simulink library "tramontina_database_curtislib"  (R2023a)
settings: Solver=VariableStepAuto  StartTime=0.0  StopTime=10.0  RelTol=1e-3
libraries: canmsglib x22, simulink x1
settings Model: Creator=matlab.cut  LastModifiedBy=matlab.cut

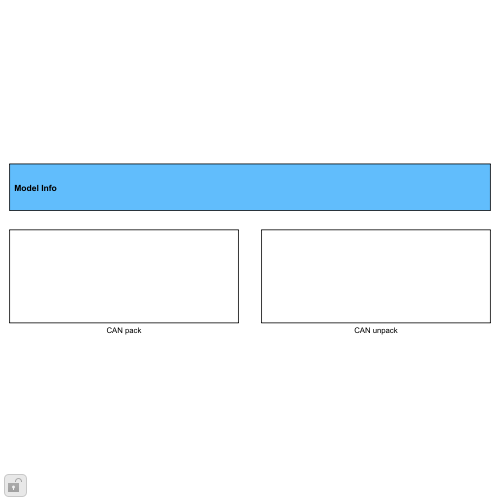
[thumbnail: Simulink's stored preview of the top-level diagram]
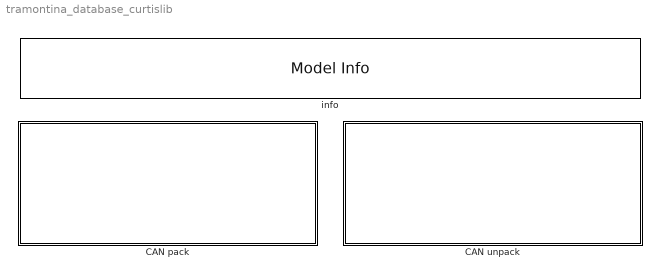
== system tramontina_database_curtislib ==
  CAN pack : Subsystem
  CAN unpack : Subsystem
  info : simulink/Model-Wide Utilities/Model Info  Frame=on  DisplayStringWithTags=SPEEDGOAT CAN Database Library for: tramontina_database_curtis  HorizontalTextAlignment=Left  LeftAlignmentValue=0.01

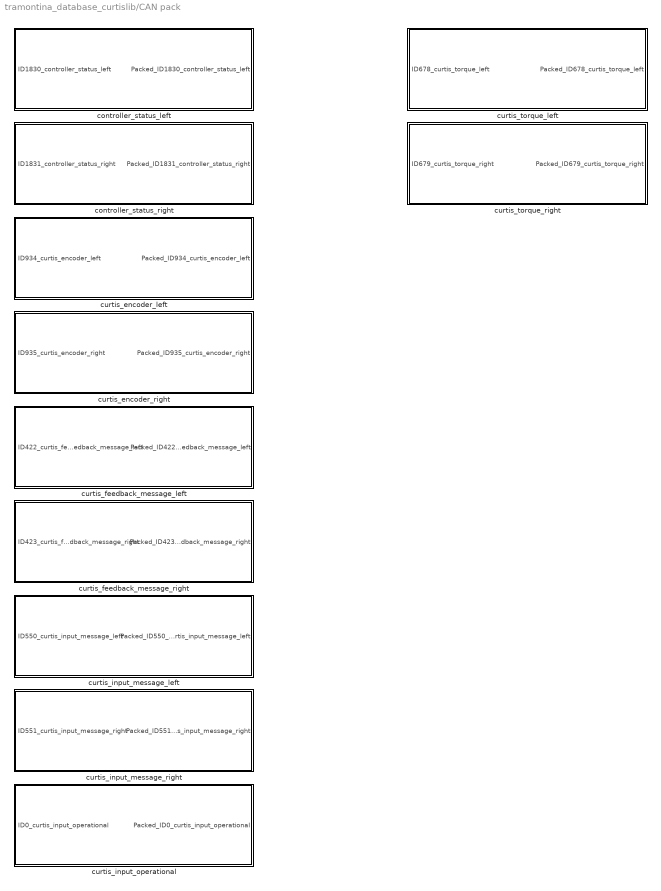
== system tramontina_database_curtislib/CAN pack ==
  controller_status_left : Subsystem
  controller_status_right : Subsystem
  curtis_encoder_left : Subsystem
  curtis_encoder_right : Subsystem
  curtis_feedback_message_left : Subsystem
  curtis_feedback_message_right : Subsystem
  curtis_input_message_left : Subsystem
  curtis_input_message_right : Subsystem
  curtis_input_operational : Subsystem
  curtis_torque_left : Subsystem
  curtis_torque_right : Subsystem

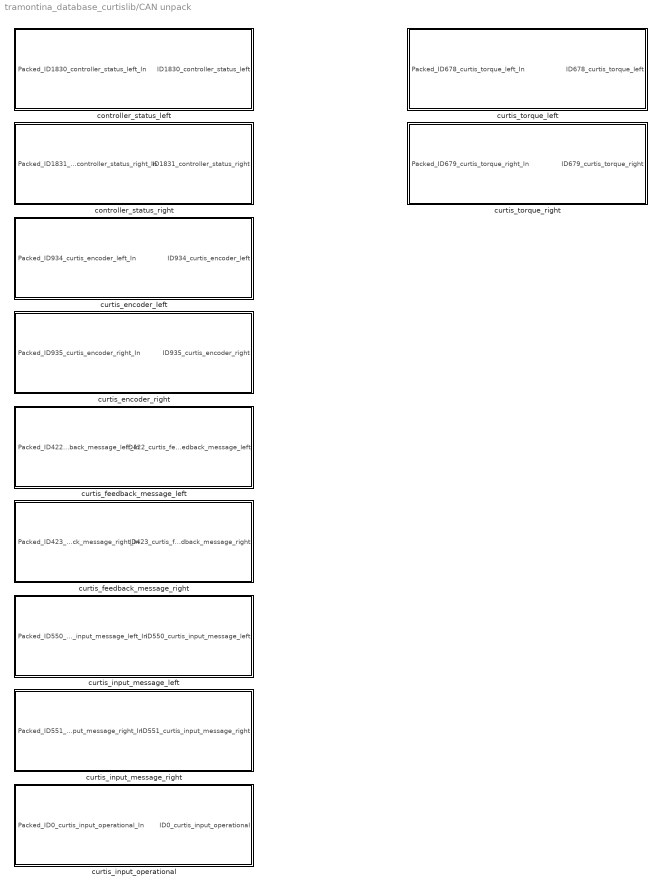
== system tramontina_database_curtislib/CAN unpack ==
  controller_status_left : Subsystem
  controller_status_right : Subsystem
  curtis_encoder_left : Subsystem
  curtis_encoder_right : Subsystem
  curtis_feedback_message_left : Subsystem
  curtis_feedback_message_right : Subsystem
  curtis_input_message_left : Subsystem
  curtis_input_message_right : Subsystem
  curtis_input_operational : Subsystem
  curtis_torque_left : Subsystem
  curtis_torque_right : Subsystem

== system tramontina_database_curtislib/CAN pack/controller_status_left ==
  In Bus Element : Inport  PortName=ID1830_controller_status_left  Element=controller_mode_left
  controller_status_left : canmsglib/CAN Pack  CANdbFile=C:\Users\matlab.cut\Desktop\matlab\dev_interno_tramontina-main\AGV-Dev-Simulink\Docs\tramontina_database_curtis.dbc  MsgList=controller_status_left  MsgName=controller_status_left  MsgIDType=Standard (11-bit identifier)  MsgIdentifier=1830  MsgLength=1  Remote=off  ApplyMinMax=off  BusOutput=on  SignalInfo={'controller_mode_left','0','8','LE','unsigned','Standard','0','1','0','0','255'}
      settings: DataFormat=manually specified signals
  Packed_ID1830_controller_status_left : Outport
  wires:
  controller_status_left/1 -> Packed_ID1830_controller_status_left/1
  In Bus Element/1 -> controller_status_left/1

== system tramontina_database_curtislib/CAN pack/controller_status_right ==
  In Bus Element : Inport  PortName=ID1831_controller_status_right  Element=controller_mode_right
  controller_status_right : canmsglib/CAN Pack  CANdbFile=C:\Users\matlab.cut\Desktop\matlab\dev_interno_tramontina-main\AGV-Dev-Simulink\Docs\tramontina_database_curtis.dbc  MsgList=controller_status_right  MsgName=controller_status_right  MsgIDType=Standard (11-bit identifier)  MsgIdentifier=1831  MsgLength=1  Remote=off  ApplyMinMax=off  BusOutput=on  SignalInfo={'controller_mode_right','0','8','LE','unsigned','Standard','0','1','0','0','255'}
      settings: DataFormat=manually specified signals
  Packed_ID1831_controller_status_right : Outport
  wires:
  controller_status_right/1 -> Packed_ID1831_controller_status_right/1
  In Bus Element/1 -> controller_status_right/1

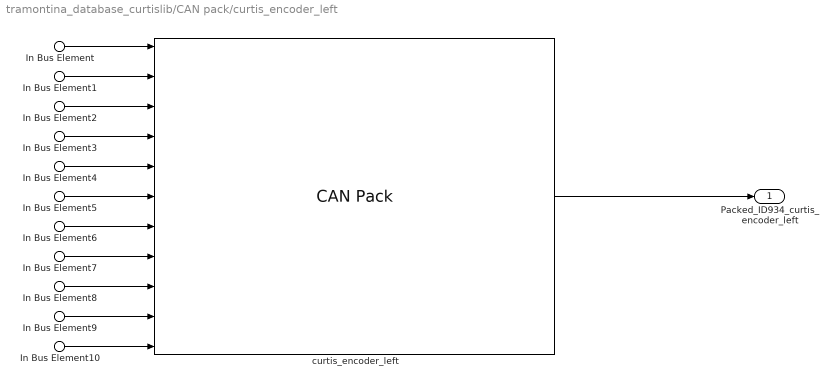
== system tramontina_database_curtislib/CAN pack/curtis_encoder_left ==
  In Bus Element : Inport  PortName=ID934_curtis_encoder_left  Element=rotor_position_left
  In Bus Element1 : Inport  PortName=ID934_curtis_encoder_left  Element=switch1
  In Bus Element2 : Inport  PortName=ID934_curtis_encoder_left  Element=switch10
  In Bus Element3 : Inport  PortName=ID934_curtis_encoder_left  Element=switch12
  In Bus Element4 : Inport  PortName=ID934_curtis_encoder_left  Element=switch13
  In Bus Element5 : Inport  PortName=ID934_curtis_encoder_left  Element=switch15
  In Bus Element6 : Inport  PortName=ID934_curtis_encoder_left  Element=switch18
  In Bus Element7 : Inport  PortName=ID934_curtis_encoder_left  Element=switch6
  In Bus Element8 : Inport  PortName=ID934_curtis_encoder_left  Element=switch7
  In Bus Element9 : Inport  PortName=ID934_curtis_encoder_left  Element=switch8
  In Bus Element10 : Inport  PortName=ID934_curtis_encoder_left  Element=switch9
  curtis_encoder_left : canmsglib/CAN Pack  CANdbFile=C:\Users\matlab.cut\Desktop\matlab\dev_interno_tramontina-main\AGV-Dev-Simulink\Docs\tramontina_database_curtis.dbc  MsgList=curtis_encoder_left  MsgName=curtis_encoder_left  MsgIDType=Standard (11-bit identifier)  MsgIdentifier=934  MsgLength=8  Remote=off  ApplyMinMax=off  BusOutput=on  SignalInfo={'rotor_position_left','0','32','LE','signed','Standard','0','0.00024414','0','-524288','524287';'switch1','32','1','LE','unsigned','Standard','0','1','0','0','1';'switch10','41','1','LE','unsigned','Standard','0','1','0','0','1';'switch12','43','1','LE','unsigned','Standard','0','1','0','0','1';'switch13','44','1','LE','unsigned','Standard','0','1','0','0','1';'switch15','46','1','LE','unsigned','Standard','0','1','0','0','1';'switch18','49','1','LE','unsigned','Standard','0','1','0','0','1';'switch6','37','1','LE','unsigned','Standard','0','1','0','0','1';'switch7','38','1','LE','unsigned','Standard','0','1','0','0','1';'switch8','39','1','LE','unsigned','Standard','0','1','0','0','1';'switch9','40','1','LE','unsigned','Standard','0','1','0','0','1'}
      settings: DataFormat=manually specified signals
  Packed_ID934_curtis_encoder_left : Outport
  wires:
  curtis_encoder_left/1 -> Packed_ID934_curtis_encoder_left/1
  In Bus Element/1 -> curtis_encoder_left/1
  In Bus Element1/1 -> curtis_encoder_left/2
  In Bus Element2/1 -> curtis_encoder_left/3
  In Bus Element3/1 -> curtis_encoder_left/4
  In Bus Element4/1 -> curtis_encoder_left/5
  In Bus Element5/1 -> curtis_encoder_left/6
  In Bus Element6/1 -> curtis_encoder_left/7
  In Bus Element7/1 -> curtis_encoder_left/8
  In Bus Element8/1 -> curtis_encoder_left/9
  In Bus Element9/1 -> curtis_encoder_left/10
  In Bus Element10/1 -> curtis_encoder_left/11

== system tramontina_database_curtislib/CAN pack/curtis_encoder_right ==
  In Bus Element : Inport  PortName=ID935_curtis_encoder_right  Element=rotor_position_rigth
  curtis_encoder_right : canmsglib/CAN Pack  CANdbFile=C:\Users\matlab.cut\Desktop\matlab\dev_interno_tramontina-main\AGV-Dev-Simulink\Docs\tramontina_database_curtis.dbc  MsgList=curtis_encoder_right  MsgName=curtis_encoder_right  MsgIDType=Standard (11-bit identifier)  MsgIdentifier=935  MsgLength=4  Remote=off  ApplyMinMax=off  BusOutput=on  SignalInfo={'rotor_position_rigth','0','32','LE','signed','Standard','0','0.00024414','0','-524288','524287'}
      settings: DataFormat=manually specified signals
  Packed_ID935_curtis_encoder_right : Outport
  wires:
  curtis_encoder_right/1 -> Packed_ID935_curtis_encoder_right/1
  In Bus Element/1 -> curtis_encoder_right/1

== system tramontina_database_curtislib/CAN pack/curtis_feedback_message_left ==
  In Bus Element : Inport  PortName=ID422_curtis_feedback_message_left  Element=motor_current_left
  In Bus Element1 : Inport  PortName=ID422_curtis_feedback_message_left  Element=motor_rpm_left
  In Bus Element2 : Inport  PortName=ID422_curtis_feedback_message_left  Element=motor_temperature_left
  curtis_feedback_message_left : canmsglib/CAN Pack  CANdbFile=C:\Users\matlab.cut\Desktop\matlab\dev_interno_tramontina-main\AGV-Dev-Simulink\Docs\tramontina_database_curtis.dbc  MsgList=curtis_feedback_message_left  MsgName=curtis_feedback_message_left  MsgIDType=Standard (11-bit identifier)  MsgIdentifier=422  MsgLength=6  Remote=off  ApplyMinMax=off  BusOutput=on  SignalInfo={'motor_current_left','0','16','LE','unsigned','Standard','0','0.1','0','0','1000';'motor_rpm_left','16','16','LE','signed','Standard','0','1','0','-32768','32767';'motor_temperature_left','32','16','LE','signed','Standard','0','0.1','0','-100','300'}
      settings: DataFormat=manually specified signals
  Packed_ID422_curtis_feedback_message_left : Outport
  wires:
  curtis_feedback_message_left/1 -> Packed_ID422_curtis_feedback_message_left/1
  In Bus Element/1 -> curtis_feedback_message_left/1
  In Bus Element1/1 -> curtis_feedback_message_left/2
  In Bus Element2/1 -> curtis_feedback_message_left/3

== system tramontina_database_curtislib/CAN pack/curtis_feedback_message_right ==
  In Bus Element : Inport  PortName=ID423_curtis_feedback_message_right  Element=motor_current_right
  In Bus Element1 : Inport  PortName=ID423_curtis_feedback_message_right  Element=motor_rpm_right
  In Bus Element2 : Inport  PortName=ID423_curtis_feedback_message_right  Element=motor_temperature_right
  curtis_feedback_message_right : canmsglib/CAN Pack  CANdbFile=C:\Users\matlab.cut\Desktop\matlab\dev_interno_tramontina-main\AGV-Dev-Simulink\Docs\tramontina_database_curtis.dbc  MsgList=curtis_feedback_message_right  MsgName=curtis_feedback_message_right  MsgIDType=Standard (11-bit identifier)  MsgIdentifier=423  MsgLength=6  Remote=off  ApplyMinMax=off  BusOutput=on  SignalInfo={'motor_current_right','0','16','LE','unsigned','Standard','0','0.1','0','0','1000';'motor_rpm_right','16','16','LE','signed','Standard','0','1','0','-32768','32767';'motor_temperature_right','32','16','LE','signed','Standard','0','0.1','0','-100','300'}
      settings: DataFormat=manually specified signals
  Packed_ID423_curtis_feedback_message_right : Outport
  wires:
  curtis_feedback_message_right/1 -> Packed_ID423_curtis_feedback_message_right/1
  In Bus Element/1 -> curtis_feedback_message_right/1
  In Bus Element1/1 -> curtis_feedback_message_right/2
  In Bus Element2/1 -> curtis_feedback_message_right/3

== system tramontina_database_curtislib/CAN pack/curtis_input_message_left ==
  In Bus Element : Inport  PortName=ID550_curtis_input_message_left  Element=rpm_set_left
  curtis_input_message_left : canmsglib/CAN Pack  CANdbFile=C:\Users\matlab.cut\Desktop\matlab\dev_interno_tramontina-main\AGV-Dev-Simulink\Docs\tramontina_database_curtis.dbc  MsgList=curtis_input_message_left  MsgName=curtis_input_message_left  MsgIDType=Standard (11-bit identifier)  MsgIdentifier=550  MsgLength=8  Remote=off  ApplyMinMax=off  BusOutput=on  SignalInfo={'rpm_set_left','0','16','LE','signed','Standard','0','0.091553','0','-3000','3000'}
      settings: DataFormat=manually specified signals
  Packed_ID550_curtis_input_message_left : Outport
  wires:
  curtis_input_message_left/1 -> Packed_ID550_curtis_input_message_left/1
  In Bus Element/1 -> curtis_input_message_left/1

== system tramontina_database_curtislib/CAN pack/curtis_input_message_right ==
  In Bus Element : Inport  PortName=ID551_curtis_input_message_right  Element=rpm_set_right
  curtis_input_message_right : canmsglib/CAN Pack  CANdbFile=C:\Users\matlab.cut\Desktop\matlab\dev_interno_tramontina-main\AGV-Dev-Simulink\Docs\tramontina_database_curtis.dbc  MsgList=curtis_input_message_right  MsgName=curtis_input_message_right  MsgIDType=Standard (11-bit identifier)  MsgIdentifier=551  MsgLength=8  Remote=off  ApplyMinMax=off  BusOutput=on  SignalInfo={'rpm_set_right','0','16','LE','signed','Standard','0','0.091553','0','-3000','3000'}
      settings: DataFormat=manually specified signals
  Packed_ID551_curtis_input_message_right : Outport
  wires:
  curtis_input_message_right/1 -> Packed_ID551_curtis_input_message_right/1
  In Bus Element/1 -> curtis_input_message_right/1

== system tramontina_database_curtislib/CAN pack/curtis_input_operational ==
  In Bus Element : Inport  PortName=ID0_curtis_input_operational  Element=pre_operational
  curtis_input_operational : canmsglib/CAN Pack  CANdbFile=C:\Users\matlab.cut\Desktop\matlab\dev_interno_tramontina-main\AGV-Dev-Simulink\Docs\tramontina_database_curtis.dbc  MsgList=curtis_input_operational  MsgName=curtis_input_operational  MsgIDType=Standard (11-bit identifier)  MsgIdentifier=0  MsgLength=8  Remote=off  ApplyMinMax=off  BusOutput=on  SignalInfo={'pre_operational','0','8','LE','unsigned','Standard','0','1','0','-Inf','Inf'}
      settings: DataFormat=manually specified signals
  Packed_ID0_curtis_input_operational : Outport
  wires:
  curtis_input_operational/1 -> Packed_ID0_curtis_input_operational/1
  In Bus Element/1 -> curtis_input_operational/1

== system tramontina_database_curtislib/CAN pack/curtis_torque_left ==
  In Bus Element : Inport  PortName=ID678_curtis_torque_left  Element=motor_power_left
  In Bus Element1 : Inport  PortName=ID678_curtis_torque_left  Element=motor_torque_left
  curtis_torque_left : canmsglib/CAN Pack  CANdbFile=C:\Users\matlab.cut\Desktop\matlab\dev_interno_tramontina-main\AGV-Dev-Simulink\Docs\tramontina_database_curtis.dbc  MsgList=curtis_torque_left  MsgName=curtis_torque_left  MsgIDType=Standard (11-bit identifier)  MsgIdentifier=678  MsgLength=8  Remote=off  ApplyMinMax=off  BusOutput=on  SignalInfo={'motor_power_left','32','32','LE','single','Standard','0','0.1','0','-100','100';'motor_torque_left','0','32','LE','single','Standard','0','1','0','-500','500'}
      settings: DataFormat=manually specified signals
  Packed_ID678_curtis_torque_left : Outport
  wires:
  curtis_torque_left/1 -> Packed_ID678_curtis_torque_left/1
  In Bus Element/1 -> curtis_torque_left/1
  In Bus Element1/1 -> curtis_torque_left/2

== system tramontina_database_curtislib/CAN pack/curtis_torque_right ==
  In Bus Element : Inport  PortName=ID679_curtis_torque_right  Element=motor_power_rigth
  In Bus Element1 : Inport  PortName=ID679_curtis_torque_right  Element=motor_torque_rigth
  curtis_torque_right : canmsglib/CAN Pack  CANdbFile=C:\Users\matlab.cut\Desktop\matlab\dev_interno_tramontina-main\AGV-Dev-Simulink\Docs\tramontina_database_curtis.dbc  MsgList=curtis_torque_right  MsgName=curtis_torque_right  MsgIDType=Standard (11-bit identifier)  MsgIdentifier=679  MsgLength=8  Remote=off  ApplyMinMax=off  BusOutput=on  SignalInfo={'motor_power_rigth','32','32','LE','single','Standard','0','0.1','0','-100','100';'motor_torque_rigth','0','32','LE','single','Standard','0','1','0','-500','500'}
      settings: DataFormat=manually specified signals
  Packed_ID679_curtis_torque_right : Outport
  wires:
  curtis_torque_right/1 -> Packed_ID679_curtis_torque_right/1
  In Bus Element/1 -> curtis_torque_right/1
  In Bus Element1/1 -> curtis_torque_right/2

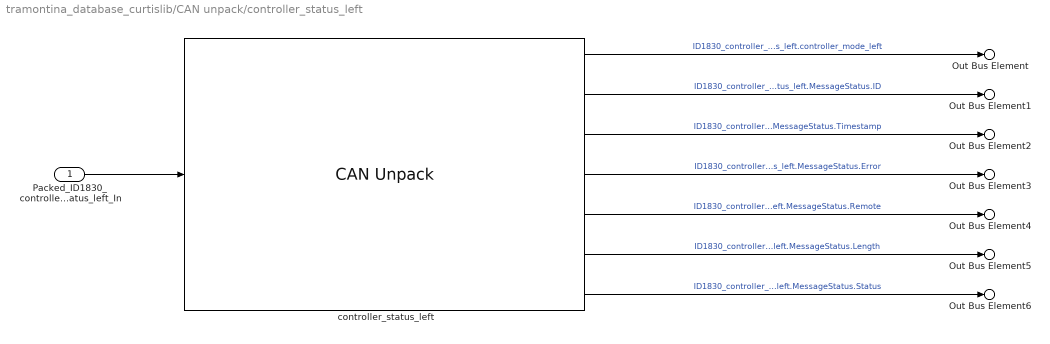
== system tramontina_database_curtislib/CAN unpack/controller_status_left ==
  Packed_ID1830_controller_status_left_In : Inport
  controller_status_left : canmsglib/CAN Unpack  CANdbFile=C:\Users\matlab.cut\Desktop\matlab\dev_interno_tramontina-main\AGV-Dev-Simulink\Docs\tramontina_database_curtis.dbc  MsgList=controller_status_left  MsgName=controller_status_left  MsgIDType=Standard (11-bit identifier)  MsgIdentifier=1830  MsgLength=1  SignalInfo={'controller_mode_left','0','8','LE','unsigned','Standard','0','1','0','0','255'}  IDPort=on  TimestampPort=on  ErrorPort=on  RemotePort=on  LengthPort=on  StatusPort=on  ApplyMinMax=off
  Out Bus Element : Outport  PortName=ID1830_controller_status_left  Element=controller_mode_left
  Out Bus Element1 : Outport  PortName=ID1830_controller_status_left  Element=MessageStatus.ID
  Out Bus Element2 : Outport  PortName=ID1830_controller_status_left  Element=MessageStatus.Timestamp
  Out Bus Element3 : Outport  PortName=ID1830_controller_status_left  Element=MessageStatus.Error
  Out Bus Element4 : Outport  PortName=ID1830_controller_status_left  Element=MessageStatus.Remote
  Out Bus Element5 : Outport  PortName=ID1830_controller_status_left  Element=MessageStatus.Length
  Out Bus Element6 : Outport  PortName=ID1830_controller_status_left  Element=MessageStatus.Status
  wires:
  Packed_ID1830_controller_status_left_In/1 -> controller_status_left/1
  controller_status_left/1 -> Out Bus Element/1  "ID1830_controller_status_left.controller_mode_left"
  controller_status_left/2 -> Out Bus Element1/1  "ID1830_controller_status_left.MessageStatus.ID"
  controller_status_left/3 -> Out Bus Element2/1  "ID1830_controller_status_left.MessageStatus.Timestamp"
  controller_status_left/4 -> Out Bus Element3/1  "ID1830_controller_status_left.MessageStatus.Error"
  controller_status_left/5 -> Out Bus Element4/1  "ID1830_controller_status_left.MessageStatus.Remote"
  controller_status_left/6 -> Out Bus Element5/1  "ID1830_controller_status_left.MessageStatus.Length"
  controller_status_left/7 -> Out Bus Element6/1  "ID1830_controller_status_left.MessageStatus.Status"

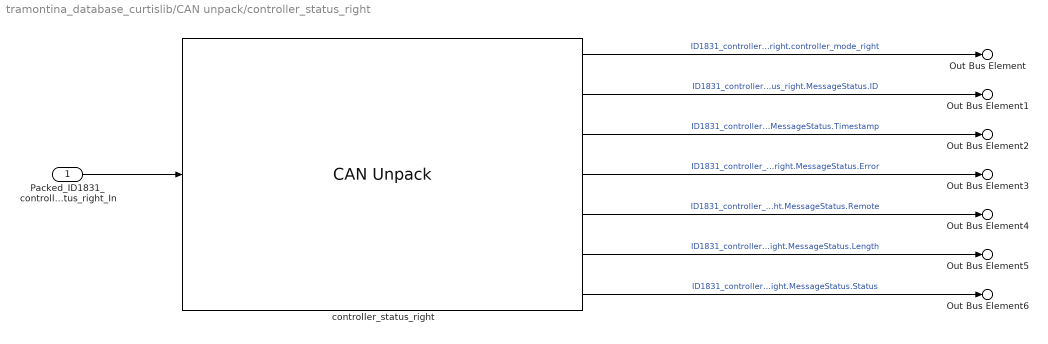
== system tramontina_database_curtislib/CAN unpack/controller_status_right ==
  Packed_ID1831_controller_status_right_In : Inport
  controller_status_right : canmsglib/CAN Unpack  CANdbFile=C:\Users\matlab.cut\Desktop\matlab\dev_interno_tramontina-main\AGV-Dev-Simulink\Docs\tramontina_database_curtis.dbc  MsgList=controller_status_right  MsgName=controller_status_right  MsgIDType=Standard (11-bit identifier)  MsgIdentifier=1831  MsgLength=1  SignalInfo={'controller_mode_right','0','8','LE','unsigned','Standard','0','1','0','0','255'}  IDPort=on  TimestampPort=on  ErrorPort=on  RemotePort=on  LengthPort=on  StatusPort=on  ApplyMinMax=off
  Out Bus Element : Outport  PortName=ID1831_controller_status_right  Element=controller_mode_right
  Out Bus Element1 : Outport  PortName=ID1831_controller_status_right  Element=MessageStatus.ID
  Out Bus Element2 : Outport  PortName=ID1831_controller_status_right  Element=MessageStatus.Timestamp
  Out Bus Element3 : Outport  PortName=ID1831_controller_status_right  Element=MessageStatus.Error
  Out Bus Element4 : Outport  PortName=ID1831_controller_status_right  Element=MessageStatus.Remote
  Out Bus Element5 : Outport  PortName=ID1831_controller_status_right  Element=MessageStatus.Length
  Out Bus Element6 : Outport  PortName=ID1831_controller_status_right  Element=MessageStatus.Status
  wires:
  Packed_ID1831_controller_status_right_In/1 -> controller_status_right/1
  controller_status_right/1 -> Out Bus Element/1  "ID1831_controller_status_right.controller_mode_right"
  controller_status_right/2 -> Out Bus Element1/1  "ID1831_controller_status_right.MessageStatus.ID"
  controller_status_right/3 -> Out Bus Element2/1  "ID1831_controller_status_right.MessageStatus.Timestamp"
  controller_status_right/4 -> Out Bus Element3/1  "ID1831_controller_status_right.MessageStatus.Error"
  controller_status_right/5 -> Out Bus Element4/1  "ID1831_controller_status_right.MessageStatus.Remote"
  controller_status_right/6 -> Out Bus Element5/1  "ID1831_controller_status_right.MessageStatus.Length"
  controller_status_right/7 -> Out Bus Element6/1  "ID1831_controller_status_right.MessageStatus.Status"

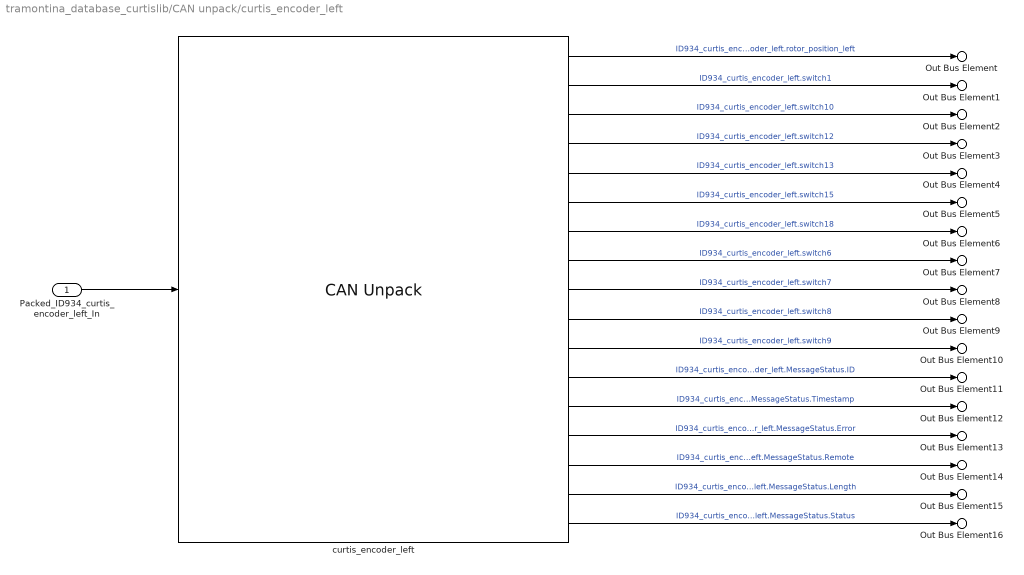
== system tramontina_database_curtislib/CAN unpack/curtis_encoder_left ==
  Packed_ID934_curtis_encoder_left_In : Inport
  curtis_encoder_left : canmsglib/CAN Unpack  CANdbFile=C:\Users\matlab.cut\Desktop\matlab\dev_interno_tramontina-main\AGV-Dev-Simulink\Docs\tramontina_database_curtis.dbc  MsgList=curtis_encoder_left  MsgName=curtis_encoder_left  MsgIDType=Standard (11-bit identifier)  MsgIdentifier=934  MsgLength=8  SignalInfo={'rotor_position_left','0','32','LE','signed','Standard','0','0.00024414','0','-524288','524287';'switch1','32','1','LE','unsigned','Standard','0','1','0','0','1';'switch10','41','1','LE','unsigned','Standard','0','1','0','0','1';'switch12','43','1','LE','unsigned','Standard','0','1','0','0','1';'switch13','44','1','LE','unsigned','Standard','0','1','0','0','1';'switch15','46','1','LE','unsigned','Standard','0','1','0','0','1';'switch18','49','1','LE','unsigned','Standard','0','1','0','0','1';'switch6','37','1','LE','unsigned','Standard','0','1','0','0','1';'switch7','38','1','LE','unsigned','Standard','0','1','0','0','1';'switch8','39','1','LE','unsigned','Standard','0','1','0','0','1';'switch9','40','1','LE','unsigned','Standard','0','1','0','0','1'}  IDPort=on  TimestampPort=on  ErrorPort=on  RemotePort=on  LengthPort=on  StatusPort=on  ApplyMinMax=off
  Out Bus Element : Outport  PortName=ID934_curtis_encoder_left  Element=rotor_position_left
  Out Bus Element1 : Outport  PortName=ID934_curtis_encoder_left  Element=switch1
  Out Bus Element2 : Outport  PortName=ID934_curtis_encoder_left  Element=switch10
  Out Bus Element3 : Outport  PortName=ID934_curtis_encoder_left  Element=switch12
  Out Bus Element4 : Outport  PortName=ID934_curtis_encoder_left  Element=switch13
  Out Bus Element5 : Outport  PortName=ID934_curtis_encoder_left  Element=switch15
  Out Bus Element6 : Outport  PortName=ID934_curtis_encoder_left  Element=switch18
  Out Bus Element7 : Outport  PortName=ID934_curtis_encoder_left  Element=switch6
  Out Bus Element8 : Outport  PortName=ID934_curtis_encoder_left  Element=switch7
  Out Bus Element9 : Outport  PortName=ID934_curtis_encoder_left  Element=switch8
  Out Bus Element10 : Outport  PortName=ID934_curtis_encoder_left  Element=switch9
  Out Bus Element11 : Outport  PortName=ID934_curtis_encoder_left  Element=MessageStatus.ID
  Out Bus Element12 : Outport  PortName=ID934_curtis_encoder_left  Element=MessageStatus.Timestamp
  Out Bus Element13 : Outport  PortName=ID934_curtis_encoder_left  Element=MessageStatus.Error
  Out Bus Element14 : Outport  PortName=ID934_curtis_encoder_left  Element=MessageStatus.Remote
  Out Bus Element15 : Outport  PortName=ID934_curtis_encoder_left  Element=MessageStatus.Length
  Out Bus Element16 : Outport  PortName=ID934_curtis_encoder_left  Element=MessageStatus.Status
  wires:
  Packed_ID934_curtis_encoder_left_In/1 -> curtis_encoder_left/1
  curtis_encoder_left/1 -> Out Bus Element/1  "ID934_curtis_encoder_left.rotor_position_left"
  curtis_encoder_left/2 -> Out Bus Element1/1  "ID934_curtis_encoder_left.switch1"
  curtis_encoder_left/3 -> Out Bus Element2/1  "ID934_curtis_encoder_left.switch10"
  curtis_encoder_left/4 -> Out Bus Element3/1  "ID934_curtis_encoder_left.switch12"
  curtis_encoder_left/5 -> Out Bus Element4/1  "ID934_curtis_encoder_left.switch13"
  curtis_encoder_left/6 -> Out Bus Element5/1  "ID934_curtis_encoder_left.switch15"
  curtis_encoder_left/7 -> Out Bus Element6/1  "ID934_curtis_encoder_left.switch18"
  curtis_encoder_left/8 -> Out Bus Element7/1  "ID934_curtis_encoder_left.switch6"
  curtis_encoder_left/9 -> Out Bus Element8/1  "ID934_curtis_encoder_left.switch7"
  curtis_encoder_left/10 -> Out Bus Element9/1  "ID934_curtis_encoder_left.switch8"
  curtis_encoder_left/11 -> Out Bus Element10/1  "ID934_curtis_encoder_left.switch9"
  curtis_encoder_left/12 -> Out Bus Element11/1  "ID934_curtis_encoder_left.MessageStatus.ID"
  curtis_encoder_left/13 -> Out Bus Element12/1  "ID934_curtis_encoder_left.MessageStatus.Timestamp"
  curtis_encoder_left/14 -> Out Bus Element13/1  "ID934_curtis_encoder_left.MessageStatus.Error"
  curtis_encoder_left/15 -> Out Bus Element14/1  "ID934_curtis_encoder_left.MessageStatus.Remote"
  curtis_encoder_left/16 -> Out Bus Element15/1  "ID934_curtis_encoder_left.MessageStatus.Length"
  curtis_encoder_left/17 -> Out Bus Element16/1  "ID934_curtis_encoder_left.MessageStatus.Status"

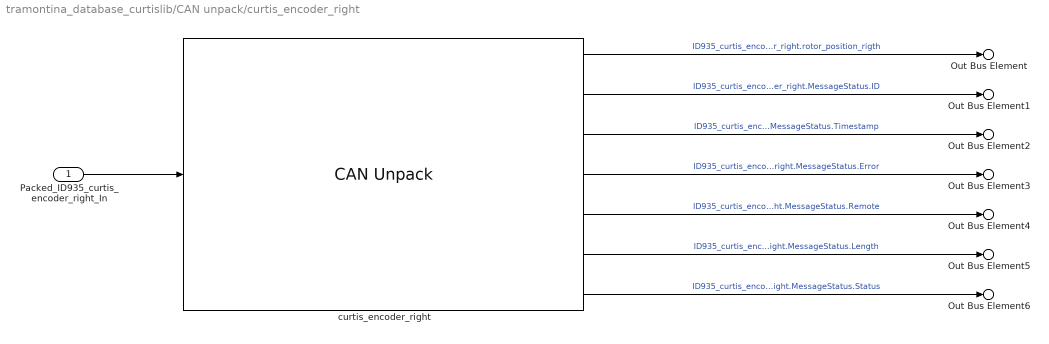
== system tramontina_database_curtislib/CAN unpack/curtis_encoder_right ==
  Packed_ID935_curtis_encoder_right_In : Inport
  curtis_encoder_right : canmsglib/CAN Unpack  CANdbFile=C:\Users\matlab.cut\Desktop\matlab\dev_interno_tramontina-main\AGV-Dev-Simulink\Docs\tramontina_database_curtis.dbc  MsgList=curtis_encoder_right  MsgName=curtis_encoder_right  MsgIDType=Standard (11-bit identifier)  MsgIdentifier=935  MsgLength=4  SignalInfo={'rotor_position_rigth','0','32','LE','signed','Standard','0','0.00024414','0','-524288','524287'}  IDPort=on  TimestampPort=on  ErrorPort=on  RemotePort=on  LengthPort=on  StatusPort=on  ApplyMinMax=off
  Out Bus Element : Outport  PortName=ID935_curtis_encoder_right  Element=rotor_position_rigth
  Out Bus Element1 : Outport  PortName=ID935_curtis_encoder_right  Element=MessageStatus.ID
  Out Bus Element2 : Outport  PortName=ID935_curtis_encoder_right  Element=MessageStatus.Timestamp
  Out Bus Element3 : Outport  PortName=ID935_curtis_encoder_right  Element=MessageStatus.Error
  Out Bus Element4 : Outport  PortName=ID935_curtis_encoder_right  Element=MessageStatus.Remote
  Out Bus Element5 : Outport  PortName=ID935_curtis_encoder_right  Element=MessageStatus.Length
  Out Bus Element6 : Outport  PortName=ID935_curtis_encoder_right  Element=MessageStatus.Status
  wires:
  Packed_ID935_curtis_encoder_right_In/1 -> curtis_encoder_right/1
  curtis_encoder_right/1 -> Out Bus Element/1  "ID935_curtis_encoder_right.rotor_position_rigth"
  curtis_encoder_right/2 -> Out Bus Element1/1  "ID935_curtis_encoder_right.MessageStatus.ID"
  curtis_encoder_right/3 -> Out Bus Element2/1  "ID935_curtis_encoder_right.MessageStatus.Timestamp"
  curtis_encoder_right/4 -> Out Bus Element3/1  "ID935_curtis_encoder_right.MessageStatus.Error"
  curtis_encoder_right/5 -> Out Bus Element4/1  "ID935_curtis_encoder_right.MessageStatus.Remote"
  curtis_encoder_right/6 -> Out Bus Element5/1  "ID935_curtis_encoder_right.MessageStatus.Length"
  curtis_encoder_right/7 -> Out Bus Element6/1  "ID935_curtis_encoder_right.MessageStatus.Status"

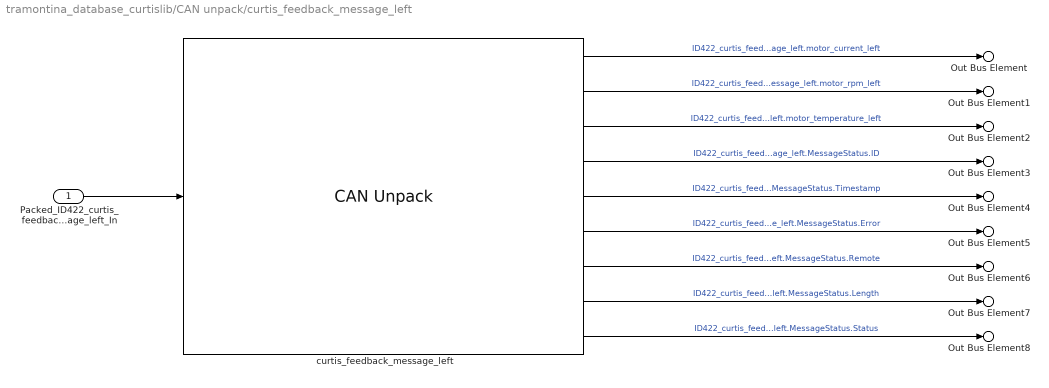
== system tramontina_database_curtislib/CAN unpack/curtis_feedback_message_left ==
  Packed_ID422_curtis_feedback_message_left_In : Inport
  curtis_feedback_message_left : canmsglib/CAN Unpack  CANdbFile=C:\Users\matlab.cut\Desktop\matlab\dev_interno_tramontina-main\AGV-Dev-Simulink\Docs\tramontina_database_curtis.dbc  MsgList=curtis_feedback_message_left  MsgName=curtis_feedback_message_left  MsgIDType=Standard (11-bit identifier)  MsgIdentifier=422  MsgLength=6  SignalInfo={'motor_current_left','0','16','LE','unsigned','Standard','0','0.1','0','0','1000';'motor_rpm_left','16','16','LE','signed','Standard','0','1','0','-32768','32767';'motor_temperature_left','32','16','LE','signed','Standard','0','0.1','0','-100','300'}  IDPort=on  TimestampPort=on  ErrorPort=on  RemotePort=on  LengthPort=on  StatusPort=on  ApplyMinMax=off
  Out Bus Element : Outport  PortName=ID422_curtis_feedback_message_left  Element=motor_current_left
  Out Bus Element1 : Outport  PortName=ID422_curtis_feedback_message_left  Element=motor_rpm_left
  Out Bus Element2 : Outport  PortName=ID422_curtis_feedback_message_left  Element=motor_temperature_left
  Out Bus Element3 : Outport  PortName=ID422_curtis_feedback_message_left  Element=MessageStatus.ID
  Out Bus Element4 : Outport  PortName=ID422_curtis_feedback_message_left  Element=MessageStatus.Timestamp
  Out Bus Element5 : Outport  PortName=ID422_curtis_feedback_message_left  Element=MessageStatus.Error
  Out Bus Element6 : Outport  PortName=ID422_curtis_feedback_message_left  Element=MessageStatus.Remote
  Out Bus Element7 : Outport  PortName=ID422_curtis_feedback_message_left  Element=MessageStatus.Length
  Out Bus Element8 : Outport  PortName=ID422_curtis_feedback_message_left  Element=MessageStatus.Status
  wires:
  Packed_ID422_curtis_feedback_message_left_In/1 -> curtis_feedback_message_left/1
  curtis_feedback_message_left/1 -> Out Bus Element/1  "ID422_curtis_feedback_message_left.motor_current_left"
  curtis_feedback_message_left/2 -> Out Bus Element1/1  "ID422_curtis_feedback_message_left.motor_rpm_left"
  curtis_feedback_message_left/3 -> Out Bus Element2/1  "ID422_curtis_feedback_message_left.motor_temperature_left"
  curtis_feedback_message_left/4 -> Out Bus Element3/1  "ID422_curtis_feedback_message_left.MessageStatus.ID"
  curtis_feedback_message_left/5 -> Out Bus Element4/1  "ID422_curtis_feedback_message_left.MessageStatus.Timestamp"
  curtis_feedback_message_left/6 -> Out Bus Element5/1  "ID422_curtis_feedback_message_left.MessageStatus.Error"
  curtis_feedback_message_left/7 -> Out Bus Element6/1  "ID422_curtis_feedback_message_left.MessageStatus.Remote"
  curtis_feedback_message_left/8 -> Out Bus Element7/1  "ID422_curtis_feedback_message_left.MessageStatus.Length"
  curtis_feedback_message_left/9 -> Out Bus Element8/1  "ID422_curtis_feedback_message_left.MessageStatus.Status"

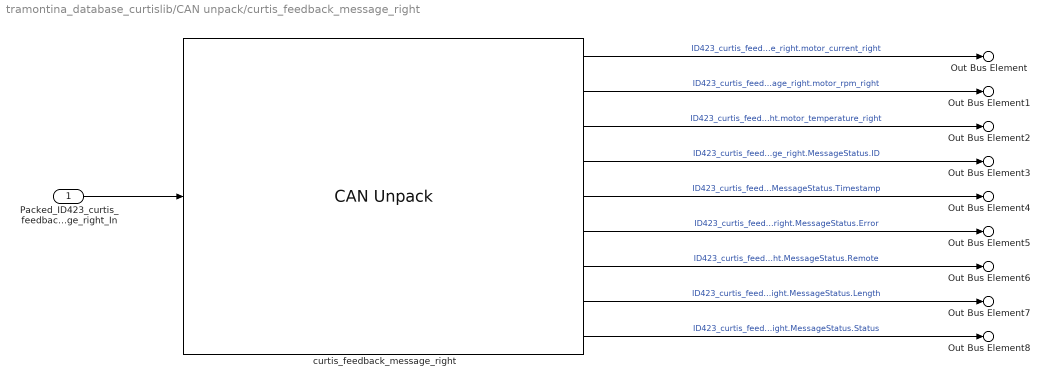
== system tramontina_database_curtislib/CAN unpack/curtis_feedback_message_right ==
  Packed_ID423_curtis_feedback_message_right_In : Inport
  curtis_feedback_message_right : canmsglib/CAN Unpack  CANdbFile=C:\Users\matlab.cut\Desktop\matlab\dev_interno_tramontina-main\AGV-Dev-Simulink\Docs\tramontina_database_curtis.dbc  MsgList=curtis_feedback_message_right  MsgName=curtis_feedback_message_right  MsgIDType=Standard (11-bit identifier)  MsgIdentifier=423  MsgLength=6  SignalInfo={'motor_current_right','0','16','LE','unsigned','Standard','0','0.1','0','0','1000';'motor_rpm_right','16','16','LE','signed','Standard','0','1','0','-32768','32767';'motor_temperature_right','32','16','LE','signed','Standard','0','0.1','0','-100','300'}  IDPort=on  TimestampPort=on  ErrorPort=on  RemotePort=on  LengthPort=on  StatusPort=on  ApplyMinMax=off
  Out Bus Element : Outport  PortName=ID423_curtis_feedback_message_right  Element=motor_current_right
  Out Bus Element1 : Outport  PortName=ID423_curtis_feedback_message_right  Element=motor_rpm_right
  Out Bus Element2 : Outport  PortName=ID423_curtis_feedback_message_right  Element=motor_temperature_right
  Out Bus Element3 : Outport  PortName=ID423_curtis_feedback_message_right  Element=MessageStatus.ID
  Out Bus Element4 : Outport  PortName=ID423_curtis_feedback_message_right  Element=MessageStatus.Timestamp
  Out Bus Element5 : Outport  PortName=ID423_curtis_feedback_message_right  Element=MessageStatus.Error
  Out Bus Element6 : Outport  PortName=ID423_curtis_feedback_message_right  Element=MessageStatus.Remote
  Out Bus Element7 : Outport  PortName=ID423_curtis_feedback_message_right  Element=MessageStatus.Length
  Out Bus Element8 : Outport  PortName=ID423_curtis_feedback_message_right  Element=MessageStatus.Status
  wires:
  Packed_ID423_curtis_feedback_message_right_In/1 -> curtis_feedback_message_right/1
  curtis_feedback_message_right/1 -> Out Bus Element/1  "ID423_curtis_feedback_message_right.motor_current_right"
  curtis_feedback_message_right/2 -> Out Bus Element1/1  "ID423_curtis_feedback_message_right.motor_rpm_right"
  curtis_feedback_message_right/3 -> Out Bus Element2/1  "ID423_curtis_feedback_message_right.motor_temperature_right"
  curtis_feedback_message_right/4 -> Out Bus Element3/1  "ID423_curtis_feedback_message_right.MessageStatus.ID"
  curtis_feedback_message_right/5 -> Out Bus Element4/1  "ID423_curtis_feedback_message_right.MessageStatus.Timestamp"
  curtis_feedback_message_right/6 -> Out Bus Element5/1  "ID423_curtis_feedback_message_right.MessageStatus.Error"
  curtis_feedback_message_right/7 -> Out Bus Element6/1  "ID423_curtis_feedback_message_right.MessageStatus.Remote"
  curtis_feedback_message_right/8 -> Out Bus Element7/1  "ID423_curtis_feedback_message_right.MessageStatus.Length"
  curtis_feedback_message_right/9 -> Out Bus Element8/1  "ID423_curtis_feedback_message_right.MessageStatus.Status"

== system tramontina_database_curtislib/CAN unpack/curtis_input_message_left ==
  Packed_ID550_curtis_input_message_left_In : Inport
  curtis_input_message_left : canmsglib/CAN Unpack  CANdbFile=C:\Users\matlab.cut\Desktop\matlab\dev_interno_tramontina-main\AGV-Dev-Simulink\Docs\tramontina_database_curtis.dbc  MsgList=curtis_input_message_left  MsgName=curtis_input_message_left  MsgIDType=Standard (11-bit identifier)  MsgIdentifier=550  MsgLength=8  SignalInfo={'rpm_set_left','0','16','LE','signed','Standard','0','0.091553','0','-3000','3000'}  IDPort=on  TimestampPort=on  ErrorPort=on  RemotePort=on  LengthPort=on  StatusPort=on  ApplyMinMax=off
  Out Bus Element : Outport  PortName=ID550_curtis_input_message_left  Element=rpm_set_left
  Out Bus Element1 : Outport  PortName=ID550_curtis_input_message_left  Element=MessageStatus.ID
  Out Bus Element2 : Outport  PortName=ID550_curtis_input_message_left  Element=MessageStatus.Timestamp
  Out Bus Element3 : Outport  PortName=ID550_curtis_input_message_left  Element=MessageStatus.Error
  Out Bus Element4 : Outport  PortName=ID550_curtis_input_message_left  Element=MessageStatus.Remote
  Out Bus Element5 : Outport  PortName=ID550_curtis_input_message_left  Element=MessageStatus.Length
  Out Bus Element6 : Outport  PortName=ID550_curtis_input_message_left  Element=MessageStatus.Status
  wires:
  Packed_ID550_curtis_input_message_left_In/1 -> curtis_input_message_left/1
  curtis_input_message_left/1 -> Out Bus Element/1  "ID550_curtis_input_message_left.rpm_set_left"
  curtis_input_message_left/2 -> Out Bus Element1/1  "ID550_curtis_input_message_left.MessageStatus.ID"
  curtis_input_message_left/3 -> Out Bus Element2/1  "ID550_curtis_input_message_left.MessageStatus.Timestamp"
  curtis_input_message_left/4 -> Out Bus Element3/1  "ID550_curtis_input_message_left.MessageStatus.Error"
  curtis_input_message_left/5 -> Out Bus Element4/1  "ID550_curtis_input_message_left.MessageStatus.Remote"
  curtis_input_message_left/6 -> Out Bus Element5/1  "ID550_curtis_input_message_left.MessageStatus.Length"
  curtis_input_message_left/7 -> Out Bus Element6/1  "ID550_curtis_input_message_left.MessageStatus.Status"

== system tramontina_database_curtislib/CAN unpack/curtis_input_message_right ==
  Packed_ID551_curtis_input_message_right_In : Inport
  curtis_input_message_right : canmsglib/CAN Unpack  CANdbFile=C:\Users\matlab.cut\Desktop\matlab\dev_interno_tramontina-main\AGV-Dev-Simulink\Docs\tramontina_database_curtis.dbc  MsgList=curtis_input_message_right  MsgName=curtis_input_message_right  MsgIDType=Standard (11-bit identifier)  MsgIdentifier=551  MsgLength=8  SignalInfo={'rpm_set_right','0','16','LE','signed','Standard','0','0.091553','0','-3000','3000'}  IDPort=on  TimestampPort=on  ErrorPort=on  RemotePort=on  LengthPort=on  StatusPort=on  ApplyMinMax=off
  Out Bus Element : Outport  PortName=ID551_curtis_input_message_right  Element=rpm_set_right
  Out Bus Element1 : Outport  PortName=ID551_curtis_input_message_right  Element=MessageStatus.ID
  Out Bus Element2 : Outport  PortName=ID551_curtis_input_message_right  Element=MessageStatus.Timestamp
  Out Bus Element3 : Outport  PortName=ID551_curtis_input_message_right  Element=MessageStatus.Error
  Out Bus Element4 : Outport  PortName=ID551_curtis_input_message_right  Element=MessageStatus.Remote
  Out Bus Element5 : Outport  PortName=ID551_curtis_input_message_right  Element=MessageStatus.Length
  Out Bus Element6 : Outport  PortName=ID551_curtis_input_message_right  Element=MessageStatus.Status
  wires:
  Packed_ID551_curtis_input_message_right_In/1 -> curtis_input_message_right/1
  curtis_input_message_right/1 -> Out Bus Element/1  "ID551_curtis_input_message_right.rpm_set_right"
  curtis_input_message_right/2 -> Out Bus Element1/1  "ID551_curtis_input_message_right.MessageStatus.ID"
  curtis_input_message_right/3 -> Out Bus Element2/1  "ID551_curtis_input_message_right.MessageStatus.Timestamp"
  curtis_input_message_right/4 -> Out Bus Element3/1  "ID551_curtis_input_message_right.MessageStatus.Error"
  curtis_input_message_right/5 -> Out Bus Element4/1  "ID551_curtis_input_message_right.MessageStatus.Remote"
  curtis_input_message_right/6 -> Out Bus Element5/1  "ID551_curtis_input_message_right.MessageStatus.Length"
  curtis_input_message_right/7 -> Out Bus Element6/1  "ID551_curtis_input_message_right.MessageStatus.Status"

== system tramontina_database_curtislib/CAN unpack/curtis_input_operational ==
  Packed_ID0_curtis_input_operational_In : Inport
  curtis_input_operational : canmsglib/CAN Unpack  CANdbFile=C:\Users\matlab.cut\Desktop\matlab\dev_interno_tramontina-main\AGV-Dev-Simulink\Docs\tramontina_database_curtis.dbc  MsgList=curtis_input_operational  MsgName=curtis_input_operational  MsgIDType=Standard (11-bit identifier)  MsgIdentifier=0  MsgLength=8  SignalInfo={'pre_operational','0','8','LE','unsigned','Standard','0','1','0','-Inf','Inf'}  IDPort=on  TimestampPort=on  ErrorPort=on  RemotePort=on  LengthPort=on  StatusPort=on  ApplyMinMax=off
  Out Bus Element : Outport  PortName=ID0_curtis_input_operational  Element=pre_operational
  Out Bus Element1 : Outport  PortName=ID0_curtis_input_operational  Element=MessageStatus.ID
  Out Bus Element2 : Outport  PortName=ID0_curtis_input_operational  Element=MessageStatus.Timestamp
  Out Bus Element3 : Outport  PortName=ID0_curtis_input_operational  Element=MessageStatus.Error
  Out Bus Element4 : Outport  PortName=ID0_curtis_input_operational  Element=MessageStatus.Remote
  Out Bus Element5 : Outport  PortName=ID0_curtis_input_operational  Element=MessageStatus.Length
  Out Bus Element6 : Outport  PortName=ID0_curtis_input_operational  Element=MessageStatus.Status
  wires:
  Packed_ID0_curtis_input_operational_In/1 -> curtis_input_operational/1
  curtis_input_operational/1 -> Out Bus Element/1  "ID0_curtis_input_operational.pre_operational"
  curtis_input_operational/2 -> Out Bus Element1/1  "ID0_curtis_input_operational.MessageStatus.ID"
  curtis_input_operational/3 -> Out Bus Element2/1  "ID0_curtis_input_operational.MessageStatus.Timestamp"
  curtis_input_operational/4 -> Out Bus Element3/1  "ID0_curtis_input_operational.MessageStatus.Error"
  curtis_input_operational/5 -> Out Bus Element4/1  "ID0_curtis_input_operational.MessageStatus.Remote"
  curtis_input_operational/6 -> Out Bus Element5/1  "ID0_curtis_input_operational.MessageStatus.Length"
  curtis_input_operational/7 -> Out Bus Element6/1  "ID0_curtis_input_operational.MessageStatus.Status"

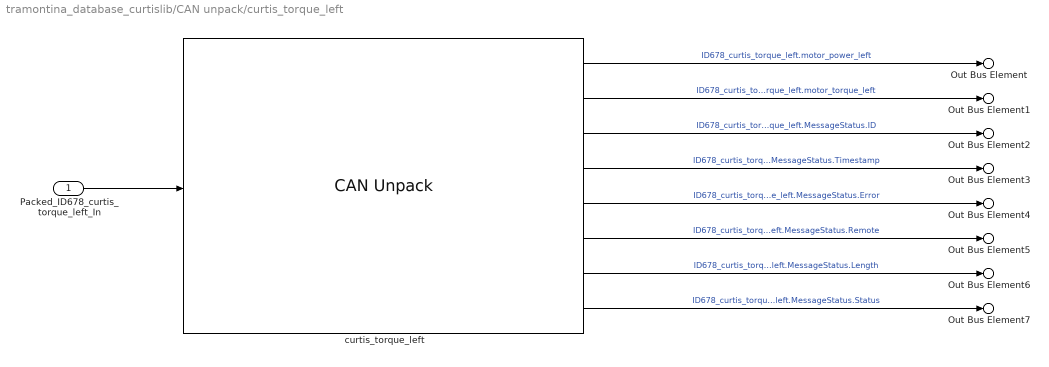
== system tramontina_database_curtislib/CAN unpack/curtis_torque_left ==
  Packed_ID678_curtis_torque_left_In : Inport
  curtis_torque_left : canmsglib/CAN Unpack  CANdbFile=C:\Users\matlab.cut\Desktop\matlab\dev_interno_tramontina-main\AGV-Dev-Simulink\Docs\tramontina_database_curtis.dbc  MsgList=curtis_torque_left  MsgName=curtis_torque_left  MsgIDType=Standard (11-bit identifier)  MsgIdentifier=678  MsgLength=8  SignalInfo={'motor_power_left','32','32','LE','single','Standard','0','0.1','0','-100','100';'motor_torque_left','0','32','LE','single','Standard','0','1','0','-500','500'}  IDPort=on  TimestampPort=on  ErrorPort=on  RemotePort=on  LengthPort=on  StatusPort=on  ApplyMinMax=off
  Out Bus Element : Outport  PortName=ID678_curtis_torque_left  Element=motor_power_left
  Out Bus Element1 : Outport  PortName=ID678_curtis_torque_left  Element=motor_torque_left
  Out Bus Element2 : Outport  PortName=ID678_curtis_torque_left  Element=MessageStatus.ID
  Out Bus Element3 : Outport  PortName=ID678_curtis_torque_left  Element=MessageStatus.Timestamp
  Out Bus Element4 : Outport  PortName=ID678_curtis_torque_left  Element=MessageStatus.Error
  Out Bus Element5 : Outport  PortName=ID678_curtis_torque_left  Element=MessageStatus.Remote
  Out Bus Element6 : Outport  PortName=ID678_curtis_torque_left  Element=MessageStatus.Length
  Out Bus Element7 : Outport  PortName=ID678_curtis_torque_left  Element=MessageStatus.Status
  wires:
  Packed_ID678_curtis_torque_left_In/1 -> curtis_torque_left/1
  curtis_torque_left/1 -> Out Bus Element/1  "ID678_curtis_torque_left.motor_power_left"
  curtis_torque_left/2 -> Out Bus Element1/1  "ID678_curtis_torque_left.motor_torque_left"
  curtis_torque_left/3 -> Out Bus Element2/1  "ID678_curtis_torque_left.MessageStatus.ID"
  curtis_torque_left/4 -> Out Bus Element3/1  "ID678_curtis_torque_left.MessageStatus.Timestamp"
  curtis_torque_left/5 -> Out Bus Element4/1  "ID678_curtis_torque_left.MessageStatus.Error"
  curtis_torque_left/6 -> Out Bus Element5/1  "ID678_curtis_torque_left.MessageStatus.Remote"
  curtis_torque_left/7 -> Out Bus Element6/1  "ID678_curtis_torque_left.MessageStatus.Length"
  curtis_torque_left/8 -> Out Bus Element7/1  "ID678_curtis_torque_left.MessageStatus.Status"

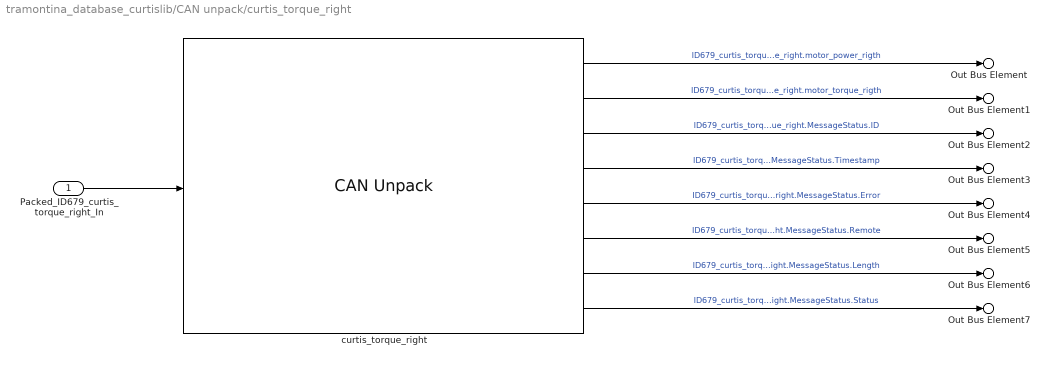
== system tramontina_database_curtislib/CAN unpack/curtis_torque_right ==
  Packed_ID679_curtis_torque_right_In : Inport
  curtis_torque_right : canmsglib/CAN Unpack  CANdbFile=C:\Users\matlab.cut\Desktop\matlab\dev_interno_tramontina-main\AGV-Dev-Simulink\Docs\tramontina_database_curtis.dbc  MsgList=curtis_torque_right  MsgName=curtis_torque_right  MsgIDType=Standard (11-bit identifier)  MsgIdentifier=679  MsgLength=8  SignalInfo={'motor_power_rigth','32','32','LE','single','Standard','0','0.1','0','-100','100';'motor_torque_rigth','0','32','LE','single','Standard','0','1','0','-500','500'}  IDPort=on  TimestampPort=on  ErrorPort=on  RemotePort=on  LengthPort=on  StatusPort=on  ApplyMinMax=off
  Out Bus Element : Outport  PortName=ID679_curtis_torque_right  Element=motor_power_rigth
  Out Bus Element1 : Outport  PortName=ID679_curtis_torque_right  Element=motor_torque_rigth
  Out Bus Element2 : Outport  PortName=ID679_curtis_torque_right  Element=MessageStatus.ID
  Out Bus Element3 : Outport  PortName=ID679_curtis_torque_right  Element=MessageStatus.Timestamp
  Out Bus Element4 : Outport  PortName=ID679_curtis_torque_right  Element=MessageStatus.Error
  Out Bus Element5 : Outport  PortName=ID679_curtis_torque_right  Element=MessageStatus.Remote
  Out Bus Element6 : Outport  PortName=ID679_curtis_torque_right  Element=MessageStatus.Length
  Out Bus Element7 : Outport  PortName=ID679_curtis_torque_right  Element=MessageStatus.Status
  wires:
  Packed_ID679_curtis_torque_right_In/1 -> curtis_torque_right/1
  curtis_torque_right/1 -> Out Bus Element/1  "ID679_curtis_torque_right.motor_power_rigth"
  curtis_torque_right/2 -> Out Bus Element1/1  "ID679_curtis_torque_right.motor_torque_rigth"
  curtis_torque_right/3 -> Out Bus Element2/1  "ID679_curtis_torque_right.MessageStatus.ID"
  curtis_torque_right/4 -> Out Bus Element3/1  "ID679_curtis_torque_right.MessageStatus.Timestamp"
  curtis_torque_right/5 -> Out Bus Element4/1  "ID679_curtis_torque_right.MessageStatus.Error"
  curtis_torque_right/6 -> Out Bus Element5/1  "ID679_curtis_torque_right.MessageStatus.Remote"
  curtis_torque_right/7 -> Out Bus Element6/1  "ID679_curtis_torque_right.MessageStatus.Length"
  curtis_torque_right/8 -> Out Bus Element7/1  "ID679_curtis_torque_right.MessageStatus.Status"
